simulink model "APP_MyApplication"  (R2018b)
settings: Solver=VariableStepDiscrete  StartTime=0.0  StopTime=10  RelTol=1e-3
PreLoadFcn:
  | if(exist('MBDS_ModelCallback', 'file')), MBDS_ModelCallback('PreLoad'); end;
PostLoadFcn:
  | if(exist('MBDS_ModelCallback', 'file')), MBDS_ModelCallback('PostLoad'); end;
InitFcn:
  | if(exist('MBDS_ModelCallback', 'file')), MBDS_ModelCallback('Init'); end;
StartFcn:
  | if(exist('MBDS_ModelCallback', 'file')), MBDS_ModelCallback('Start'); end;
StopFcn:
  | if(exist('MBDS_ModelCallback', 'file')), MBDS_ModelCallback('Stop'); end;
undefined symbols (not defined in the file): sigbuilder_block, Ts
libraries: KIBES_Signal x499, simulink x8
(part 6 of 10)

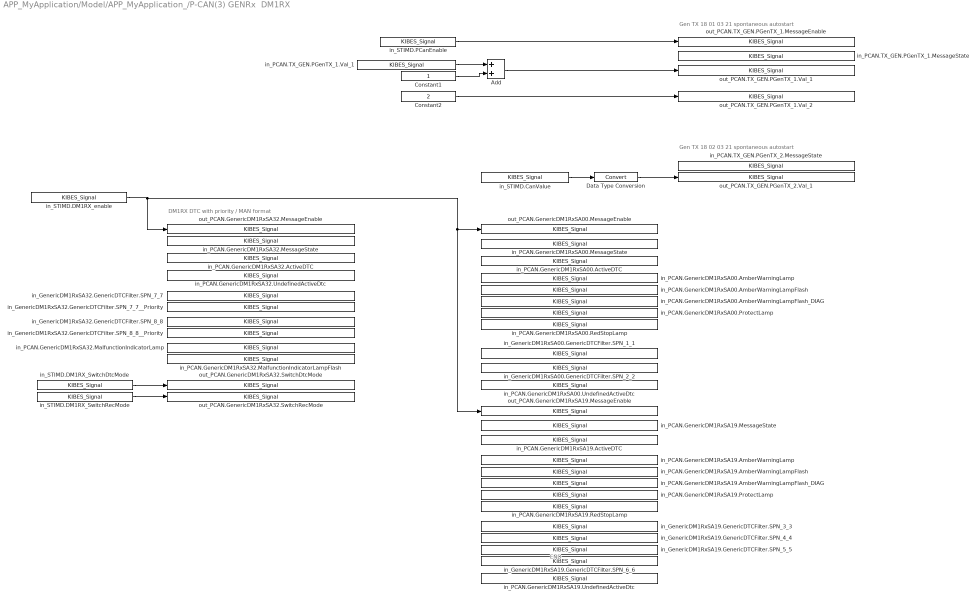
== system APP_MyApplication/Model/APP_MyApplication_/P-CAN(3) GENRx  DM1RX ==
  note: END
  note: Gen TX 18 01 03 21 spontaneous autostart
  note: Gen TX 18 02 03 21 spontaneous autostart
  note: DM1RX DTC with priority / MAN format
  Add : Sum  InitFcn=|  OutDataTypeStr=Inherit: Inherit via back propagation
      | if(exist('MBDS_BlockCallback', 'file'))
      |    MBDS_BlockCallback('Update', gcb);  
      | end
      settings: AttributesFormatString=Saturate: %<SaturateOnIntegerOverflow>
  Constant1 : Constant  InitFcn=|  OutDataTypeStr=uint8
      | if(exist('MBDS_BlockCallback', 'file'))
      |    MBDS_BlockCallback('Update', gcb);  
      | end
  Constant2 : Constant  InitFcn=|  Value=2  OutDataTypeStr=uint8
      | if(exist('MBDS_BlockCallback', 'file'))
      |    MBDS_BlockCallback('Update', gcb);  
      | end
  Data Type Conversion : DataTypeConversion  InitFcn=|  SaturateOnIntegerOverflow=on
      | try
      |    MBDS_BlockCallback('Update', gcb);
      | end
      settings: AttributesFormatString=Saturate: %<SaturateOnIntegerOverflow>
  in_GenericDM1RxSA00.GenericDTCFilter.SPN_1_1 : KIBES_Signal/KIBES_Signal  MBDS_LibraryBlock=on  DatabaseKey=293  SignalName=GenericDM1RxSA00.GenericDTCFilter.SPN_1_1  SymbolName=GenericDM1RxSA00_GenericDTCFilter_SPN_1_1_000293  DataType=boolean  Init=0  Slope=1  Bias=0  DataSize=1  fpDataType=boolean  BlockIOType=Inport  DeviceType=0
  in_GenericDM1RxSA00.GenericDTCFilter.SPN_2_2 : KIBES_Signal/KIBES_Signal  MBDS_LibraryBlock=on  DatabaseKey=294  SignalName=GenericDM1RxSA00.GenericDTCFilter.SPN_2_2  SymbolName=GenericDM1RxSA00_GenericDTCFilter_SPN_2_2_000294  DataType=boolean  Init=0  Slope=1  Bias=0  DataSize=1  fpDataType=boolean  BlockIOType=Inport  DeviceType=0
  in_GenericDM1RxSA19.GenericDTCFilter.SPN_3_3 : KIBES_Signal/KIBES_Signal  MBDS_LibraryBlock=on  DatabaseKey=290  SignalName=GenericDM1RxSA19.GenericDTCFilter.SPN_3_3  SymbolName=GenericDM1RxSA19_GenericDTCFilter_SPN_3_3_000290  DataType=boolean  Init=0  Slope=1  Bias=0  DataSize=1  fpDataType=boolean  BlockIOType=Inport  DeviceType=0
  in_GenericDM1RxSA19.GenericDTCFilter.SPN_4_4 : KIBES_Signal/KIBES_Signal  MBDS_LibraryBlock=on  DatabaseKey=291  SignalName=GenericDM1RxSA19.GenericDTCFilter.SPN_4_4  SymbolName=GenericDM1RxSA19_GenericDTCFilter_SPN_4_4_000291  DataType=boolean  Init=0  Slope=1  Bias=0  DataSize=1  fpDataType=boolean  BlockIOType=Inport  DeviceType=0
  in_GenericDM1RxSA19.GenericDTCFilter.SPN_5_5 : KIBES_Signal/KIBES_Signal  MBDS_LibraryBlock=on  DatabaseKey=296  SignalName=GenericDM1RxSA19.GenericDTCFilter.SPN_5_5  SymbolName=GenericDM1RxSA19_GenericDTCFilter_SPN_5_5_000296  DataType=boolean  Init=0  Slope=1  Bias=0  DataSize=1  fpDataType=boolean  BlockIOType=Inport  DeviceType=0
  in_GenericDM1RxSA19.GenericDTCFilter.SPN_6_6 : KIBES_Signal/KIBES_Signal  MBDS_LibraryBlock=on  DatabaseKey=303  SignalName=GenericDM1RxSA19.GenericDTCFilter.SPN_6_6  SymbolName=GenericDM1RxSA19_GenericDTCFilter_SPN_6_6_000303  DataType=boolean  Init=0  Slope=1  Bias=0  DataSize=1  fpDataType=boolean  BlockIOType=Inport  DeviceType=0
  in_GenericDM1RxSA32.GenericDTCFilter.SPN_7_7 : KIBES_Signal/KIBES_Signal  MBDS_LibraryBlock=on  DatabaseKey=592  SignalName=GenericDM1RxSA32.GenericDTCFilter.SPN_7_7  SymbolName=GenericDM1RxSA32_GenericDTCFilter_SPN_7_7_000592  DataType=boolean  Init=0  Slope=1  Bias=0  DataSize=1  fpDataType=boolean  BlockIOType=Inport  DeviceType=0
  in_GenericDM1RxSA32.GenericDTCFilter.SPN_7_7__Priority : KIBES_Signal/KIBES_Signal  MBDS_LibraryBlock=on  DatabaseKey=593  SignalName=GenericDM1RxSA32.GenericDTCFilter.SPN_7_7__Priority  SymbolName=GenericDM1RxSA32_GenericDTCFilter_SPN_7_7__Priority_000593  DataType=uint8  Init=0  Slope=1  Bias=0  DataSize=1  fpDataType=uint8  BlockIOType=Inport  DeviceType=0
  in_GenericDM1RxSA32.GenericDTCFilter.SPN_8_8 : KIBES_Signal/KIBES_Signal  MBDS_LibraryBlock=on  DatabaseKey=594  SignalName=GenericDM1RxSA32.GenericDTCFilter.SPN_8_8  SymbolName=GenericDM1RxSA32_GenericDTCFilter_SPN_8_8_000594  DataType=boolean  Init=0  Slope=1  Bias=0  DataSize=1  fpDataType=boolean  BlockIOType=Inport  DeviceType=0
  in_GenericDM1RxSA32.GenericDTCFilter.SPN_8_8__Priority : KIBES_Signal/KIBES_Signal  MBDS_LibraryBlock=on  DatabaseKey=595  SignalName=GenericDM1RxSA32.GenericDTCFilter.SPN_8_8__Priority  SymbolName=GenericDM1RxSA32_GenericDTCFilter_SPN_8_8__Priority_000595  DataType=uint8  Init=0  Slope=1  Bias=0  DataSize=1  fpDataType=uint8  BlockIOType=Inport  DeviceType=0
  in_PCAN.GenericDM1RxSA00.ActiveDTC : KIBES_Signal/KIBES_Signal  MBDS_LibraryBlock=on  DatabaseKey=274  SignalName=PCAN.GenericDM1RxSA00.ActiveDTC  SymbolName=PCAN_GenericDM1RxSA00_ActiveDTC_000274  DataType=boolean  Init=0  Slope=1  Bias=0  DataSize=1  fpDataType=boolean  BlockIOType=Inport  DeviceType=0
  in_PCAN.GenericDM1RxSA00.AmberWarningLamp : KIBES_Signal/KIBES_Signal  MBDS_LibraryBlock=on  DatabaseKey=275  SignalName=PCAN.GenericDM1RxSA00.AmberWarningLamp  SymbolName=PCAN_GenericDM1RxSA00_AmberWarningLamp_000275  DataType=boolean  Init=0  Slope=1  Bias=0  DataSize=1  fpDataType=boolean  BlockIOType=Inport  DeviceType=0
  in_PCAN.GenericDM1RxSA00.AmberWarningLampFlash : KIBES_Signal/KIBES_Signal  MBDS_LibraryBlock=on  DatabaseKey=276  SignalName=PCAN.GenericDM1RxSA00.AmberWarningLampFlash  SymbolName=PCAN_GenericDM1RxSA00_AmberWarningLampFlash_000276  DataType=uint8  Init=0  Slope=1  Bias=0  DataSize=1  fpDataType=uint8  BlockIOType=Inport  DeviceType=0
  in_PCAN.GenericDM1RxSA00.AmberWarningLampFlash_DIAG : KIBES_Signal/KIBES_Signal  MBDS_LibraryBlock=on  DatabaseKey=277  SignalName=PCAN.GenericDM1RxSA00.AmberWarningLampFlash_DIAG  SymbolName=PCAN_GenericDM1RxSA00_AmberWarningLampFlash_DIAG_000277  DataType=uint16  Init=1  Slope=1  Bias=0  DataSize=1  fpDataType=uint16  BlockIOType=Inport  DeviceType=0
  in_PCAN.GenericDM1RxSA00.MessageState : KIBES_Signal/KIBES_Signal  MBDS_LibraryBlock=on  DatabaseKey=279  SignalName=PCAN.GenericDM1RxSA00.MessageState  SymbolName=PCAN_GenericDM1RxSA00_MessageState_000279  DataType=uint16  Init=0  Slope=1  Bias=0  DataSize=1  fpDataType=uint16  BlockIOType=Inport  DeviceType=0
  in_PCAN.GenericDM1RxSA00.ProtectLamp : KIBES_Signal/KIBES_Signal  MBDS_LibraryBlock=on  DatabaseKey=280  SignalName=PCAN.GenericDM1RxSA00.ProtectLamp  SymbolName=PCAN_GenericDM1RxSA00_ProtectLamp_000280  DataType=boolean  Init=0  Slope=1  Bias=0  DataSize=1  fpDataType=boolean  BlockIOType=Inport  DeviceType=0
  in_PCAN.GenericDM1RxSA00.RedStopLamp : KIBES_Signal/KIBES_Signal  MBDS_LibraryBlock=on  DatabaseKey=281  SignalName=PCAN.GenericDM1RxSA00.RedStopLamp  SymbolName=PCAN_GenericDM1RxSA00_RedStopLamp_000281  DataType=boolean  Init=0  Slope=1  Bias=0  DataSize=1  fpDataType=boolean  BlockIOType=Inport  DeviceType=0
  in_PCAN.GenericDM1RxSA00.UndefinedActiveDtc : KIBES_Signal/KIBES_Signal  MBDS_LibraryBlock=on  DatabaseKey=403  SignalName=PCAN.GenericDM1RxSA00.UndefinedActiveDtc  SymbolName=PCAN_GenericDM1RxSA00_UndefinedActiveDtc_000403  DataType=boolean  Init=0  Slope=1  Bias=0  DataSize=1  fpDataType=boolean  BlockIOType=Inport  DeviceType=0
  in_PCAN.GenericDM1RxSA19.ActiveDTC : KIBES_Signal/KIBES_Signal  MBDS_LibraryBlock=on  DatabaseKey=282  SignalName=PCAN.GenericDM1RxSA19.ActiveDTC  SymbolName=PCAN_GenericDM1RxSA19_ActiveDTC_000282  DataType=boolean  Init=0  Slope=1  Bias=0  DataSize=1  fpDataType=boolean  BlockIOType=Inport  DeviceType=0
  in_PCAN.GenericDM1RxSA19.AmberWarningLamp : KIBES_Signal/KIBES_Signal  MBDS_LibraryBlock=on  DatabaseKey=283  SignalName=PCAN.GenericDM1RxSA19.AmberWarningLamp  SymbolName=PCAN_GenericDM1RxSA19_AmberWarningLamp_000283  DataType=boolean  Init=0  Slope=1  Bias=0  DataSize=1  fpDataType=boolean  BlockIOType=Inport  DeviceType=0
  in_PCAN.GenericDM1RxSA19.AmberWarningLampFlash : KIBES_Signal/KIBES_Signal  MBDS_LibraryBlock=on  DatabaseKey=284  SignalName=PCAN.GenericDM1RxSA19.AmberWarningLampFlash  SymbolName=PCAN_GenericDM1RxSA19_AmberWarningLampFlash_000284  DataType=uint8  Init=0  Slope=1  Bias=0  DataSize=1  fpDataType=uint8  BlockIOType=Inport  DeviceType=0
  in_PCAN.GenericDM1RxSA19.AmberWarningLampFlash_DIAG : KIBES_Signal/KIBES_Signal  MBDS_LibraryBlock=on  DatabaseKey=285  SignalName=PCAN.GenericDM1RxSA19.AmberWarningLampFlash_DIAG  SymbolName=PCAN_GenericDM1RxSA19_AmberWarningLampFlash_DIAG_000285  DataType=uint16  Init=1  Slope=1  Bias=0  DataSize=1  fpDataType=uint16  BlockIOType=Inport  DeviceType=0
  in_PCAN.GenericDM1RxSA19.MessageState : KIBES_Signal/KIBES_Signal  MBDS_LibraryBlock=on  DatabaseKey=287  SignalName=PCAN.GenericDM1RxSA19.MessageState  SymbolName=PCAN_GenericDM1RxSA19_MessageState_000287  DataType=uint16  Init=0  Slope=1  Bias=0  DataSize=1  fpDataType=uint16  BlockIOType=Inport  DeviceType=0
  in_PCAN.GenericDM1RxSA19.ProtectLamp : KIBES_Signal/KIBES_Signal  MBDS_LibraryBlock=on  DatabaseKey=288  SignalName=PCAN.GenericDM1RxSA19.ProtectLamp  SymbolName=PCAN_GenericDM1RxSA19_ProtectLamp_000288  DataType=boolean  Init=0  Slope=1  Bias=0  DataSize=1  fpDataType=boolean  BlockIOType=Inport  DeviceType=0
  in_PCAN.GenericDM1RxSA19.RedStopLamp : KIBES_Signal/KIBES_Signal  MBDS_LibraryBlock=on  DatabaseKey=289  SignalName=PCAN.GenericDM1RxSA19.RedStopLamp  SymbolName=PCAN_GenericDM1RxSA19_RedStopLamp_000289  DataType=boolean  Init=0  Slope=1  Bias=0  DataSize=1  fpDataType=boolean  BlockIOType=Inport  DeviceType=0
  in_PCAN.GenericDM1RxSA19.UndefinedActiveDtc : KIBES_Signal/KIBES_Signal  MBDS_LibraryBlock=on  DatabaseKey=404  SignalName=PCAN.GenericDM1RxSA19.UndefinedActiveDtc  SymbolName=PCAN_GenericDM1RxSA19_UndefinedActiveDtc_000404  DataType=boolean  Init=0  Slope=1  Bias=0  DataSize=1  fpDataType=boolean  BlockIOType=Inport  DeviceType=0
  in_PCAN.GenericDM1RxSA32.ActiveDTC : KIBES_Signal/KIBES_Signal  MBDS_LibraryBlock=on  DatabaseKey=588  SignalName=PCAN.GenericDM1RxSA32.ActiveDTC  SymbolName=PCAN_GenericDM1RxSA32_ActiveDTC_000588  DataType=boolean  Init=0  Slope=1  Bias=0  DataSize=1  fpDataType=boolean  BlockIOType=Inport  DeviceType=0
  in_PCAN.GenericDM1RxSA32.MalfunctionIndicatorLamp : KIBES_Signal/KIBES_Signal  MBDS_LibraryBlock=on  DatabaseKey=601  SignalName=PCAN.GenericDM1RxSA32.MalfunctionIndicatorLamp  SymbolName=PCAN_GenericDM1RxSA32_MalfunctionIndicatorLamp_000601  DataType=boolean  Init=0  Slope=1  Bias=0  DataSize=1  fpDataType=boolean  BlockIOType=Inport  DeviceType=0
  in_PCAN.GenericDM1RxSA32.MalfunctionIndicatorLampFlash : KIBES_Signal/KIBES_Signal  MBDS_LibraryBlock=on  DatabaseKey=602  SignalName=PCAN.GenericDM1RxSA32.MalfunctionIndicatorLampFlash  SymbolName=PCAN_GenericDM1RxSA32_MalfunctionIndicatorLampFlash_000602  DataType=uint8  Init=0  Slope=1  Bias=0  DataSize=1  fpDataType=uint8  BlockIOType=Inport  DeviceType=0
  in_PCAN.GenericDM1RxSA32.MessageState : KIBES_Signal/KIBES_Signal  MBDS_LibraryBlock=on  DatabaseKey=590  SignalName=PCAN.GenericDM1RxSA32.MessageState  SymbolName=PCAN_GenericDM1RxSA32_MessageState_000590  DataType=uint16  Init=0  Slope=1  Bias=0  DataSize=1  fpDataType=uint16  BlockIOType=Inport  DeviceType=0
  in_PCAN.GenericDM1RxSA32.UndefinedActiveDtc : KIBES_Signal/KIBES_Signal  MBDS_LibraryBlock=on  DatabaseKey=591  SignalName=PCAN.GenericDM1RxSA32.UndefinedActiveDtc  SymbolName=PCAN_GenericDM1RxSA32_UndefinedActiveDtc_000591  DataType=boolean  Init=0  Slope=1  Bias=0  DataSize=1  fpDataType=boolean  BlockIOType=Inport  DeviceType=0
  in_PCAN.TX_GEN.PGenTX_1.MessageState : KIBES_Signal/KIBES_Signal  MBDS_LibraryBlock=on  DatabaseKey=260  SignalName=PCAN.TX_GEN.PGenTX_1.MessageState  SymbolName=PCAN_TX_GEN_PGenTX_1_MessageState_000260  DataType=uint16  Init=0  Slope=1  Bias=0  DataSize=1  fpDataType=uint16  BlockIOType=Inport  DeviceType=0
  in_PCAN.TX_GEN.PGenTX_1.Val_1 : KIBES_Signal/KIBES_Signal  MBDS_LibraryBlock=on  DatabaseKey=261  SignalName=PCAN.TX_GEN.PGenTX_1.Val_1  SymbolName=PCAN_TX_GEN_PGenTX_1_Val_1_000261  DataType=uint8  Init=0  Slope=1  Bias=0  DataSize=1  fpDataType=uint8  BlockIOType=Inport  DeviceType=0
  in_PCAN.TX_GEN.PGenTX_2.MessageState : KIBES_Signal/KIBES_Signal  MBDS_LibraryBlock=on  DatabaseKey=577  SignalName=PCAN.TX_GEN.PGenTX_2.MessageState  SymbolName=PCAN_TX_GEN_PGenTX_2_MessageState_000577  DataType=uint16  Init=0  Slope=1  Bias=0  DataSize=1  fpDataType=uint16  BlockIOType=Inport  DeviceType=0
  in_STIMD.CanValue : KIBES_Signal/KIBES_Signal  MBDS_LibraryBlock=on  DatabaseKey=585  SignalName=STIMD.CanValue  SymbolName=STIMD_CanValue_000585  DataType=int32  Init=1  Slope=1  Bias=0  DataSize=1  fpDataType=int32  BlockIOType=Inport  DeviceType=2
  in_STIMD.DM1RX_SwitchDtcMode : KIBES_Signal/KIBES_Signal  MBDS_LibraryBlock=on  DatabaseKey=599  SignalName=STIMD.DM1RX_SwitchDtcMode  SymbolName=STIMD_DM1RX_SwitchDtcMode_000599  DataType=uint8  Init=0  Slope=1  Bias=0  DataSize=1  fpDataType=uint8  BlockIOType=Inport  DeviceType=2
  in_STIMD.DM1RX_SwitchRecMode : KIBES_Signal/KIBES_Signal  MBDS_LibraryBlock=on  DatabaseKey=600  SignalName=STIMD.DM1RX_SwitchRecMode  SymbolName=STIMD_DM1RX_SwitchRecMode_000600  DataType=uint8  Init=1  Slope=1  Bias=0  DataSize=1  fpDataType=uint8  BlockIOType=Inport  DeviceType=2
  in_STIMD.DM1RX_enable : KIBES_Signal/KIBES_Signal  MBDS_LibraryBlock=on  DatabaseKey=598  SignalName=STIMD.DM1RX_enable  SymbolName=STIMD_DM1RX_enable_000598  DataType=boolean  Init=1  Slope=1  Bias=0  DataSize=1  fpDataType=boolean  BlockIOType=Inport  DeviceType=2
  in_STIMD.PCanEnable : KIBES_Signal/KIBES_Signal  MBDS_LibraryBlock=on  DatabaseKey=497  SignalName=STIMD.PCanEnable  SymbolName=STIMD_PCanEnable_000497  DataType=boolean  Init=0  Slope=1  Bias=0  DataSize=1  fpDataType=boolean  BlockIOType=Inport  DeviceType=2
  out_PCAN.GenericDM1RxSA00.MessageEnable : KIBES_Signal/KIBES_Signal  MBDS_LibraryBlock=on  DatabaseKey=278  SignalName=PCAN.GenericDM1RxSA00.MessageEnable  SymbolName=PCAN_GenericDM1RxSA00_MessageEnable_000278  DataType=boolean  Init=0  Slope=1  Bias=0  DataSize=1  fpDataType=boolean  BlockIOType=Outport  DeviceType=0
  out_PCAN.GenericDM1RxSA19.MessageEnable : KIBES_Signal/KIBES_Signal  MBDS_LibraryBlock=on  DatabaseKey=286  SignalName=PCAN.GenericDM1RxSA19.MessageEnable  SymbolName=PCAN_GenericDM1RxSA19_MessageEnable_000286  DataType=boolean  Init=0  Slope=1  Bias=0  DataSize=1  fpDataType=boolean  BlockIOType=Outport  DeviceType=0
  out_PCAN.GenericDM1RxSA32.MessageEnable : KIBES_Signal/KIBES_Signal  MBDS_LibraryBlock=on  DatabaseKey=589  SignalName=PCAN.GenericDM1RxSA32.MessageEnable  SymbolName=PCAN_GenericDM1RxSA32_MessageEnable_000589  DataType=boolean  Init=0  Slope=1  Bias=0  DataSize=1  fpDataType=boolean  BlockIOType=Outport  DeviceType=0
  out_PCAN.GenericDM1RxSA32.SwitchDtcMode : KIBES_Signal/KIBES_Signal  MBDS_LibraryBlock=on  DatabaseKey=596  SignalName=PCAN.GenericDM1RxSA32.SwitchDtcMode  SymbolName=PCAN_GenericDM1RxSA32_SwitchDtcMode_000596  DataType=uint8  Init=0  Slope=1  Bias=0  DataSize=1  fpDataType=uint8  BlockIOType=Outport  DeviceType=0
  out_PCAN.GenericDM1RxSA32.SwitchRecMode : KIBES_Signal/KIBES_Signal  MBDS_LibraryBlock=on  DatabaseKey=597  SignalName=PCAN.GenericDM1RxSA32.SwitchRecMode  SymbolName=PCAN_GenericDM1RxSA32_SwitchRecMode_000597  DataType=uint8  Init=0  Slope=1  Bias=0  DataSize=1  fpDataType=uint8  BlockIOType=Outport  DeviceType=0
  out_PCAN.TX_GEN.PGenTX_1.MessageEnable : KIBES_Signal/KIBES_Signal  MBDS_LibraryBlock=on  DatabaseKey=259  SignalName=PCAN.TX_GEN.PGenTX_1.MessageEnable  SymbolName=PCAN_TX_GEN_PGenTX_1_MessageEnable_000259  DataType=boolean  Init=0  Slope=1  Bias=0  DataSize=1  fpDataType=boolean  BlockIOType=Outport  DeviceType=0
  out_PCAN.TX_GEN.PGenTX_1.Val_1 : KIBES_Signal/KIBES_Signal  MBDS_LibraryBlock=on  DatabaseKey=261  SignalName=PCAN.TX_GEN.PGenTX_1.Val_1  SymbolName=PCAN_TX_GEN_PGenTX_1_Val_1_000261  DataType=uint8  Init=0  Slope=1  Bias=0  DataSize=1  fpDataType=uint8  BlockIOType=Outport  DeviceType=0
  out_PCAN.TX_GEN.PGenTX_1.Val_2 : KIBES_Signal/KIBES_Signal  MBDS_LibraryBlock=on  DatabaseKey=262  SignalName=PCAN.TX_GEN.PGenTX_1.Val_2  SymbolName=PCAN_TX_GEN_PGenTX_1_Val_2_000262  DataType=uint8  Init=0  Slope=1  Bias=0  DataSize=1  fpDataType=uint8  BlockIOType=Outport  DeviceType=0
  out_PCAN.TX_GEN.PGenTX_2.Val_1 : KIBES_Signal/KIBES_Signal  MBDS_LibraryBlock=on  DatabaseKey=578  SignalName=PCAN.TX_GEN.PGenTX_2.Val_1  SymbolName=PCAN_TX_GEN_PGenTX_2_Val_1_000578  DataType=uint32  Init=0  Slope=1  Bias=0  DataSize=1  fpDataType=uint32  BlockIOType=Outport  DeviceType=0
  wires:
  in_STIMD.PCanEnable/1 -> out_PCAN.TX_GEN.PGenTX_1.MessageEnable/1
  Constant2/1 -> out_PCAN.TX_GEN.PGenTX_1.Val_2/1
  in_STIMD.DM1RX_enable/1 -> out_PCAN.GenericDM1RxSA19.MessageEnable/1, out_PCAN.GenericDM1RxSA00.MessageEnable/1, out_PCAN.GenericDM1RxSA32.MessageEnable/1
  Data Type Conversion/1 -> out_PCAN.TX_GEN.PGenTX_2.Val_1/1
  in_STIMD.CanValue/1 -> Data Type Conversion/1
  in_STIMD.DM1RX_SwitchDtcMode/1 -> out_PCAN.GenericDM1RxSA32.SwitchDtcMode/1
  in_STIMD.DM1RX_SwitchRecMode/1 -> out_PCAN.GenericDM1RxSA32.SwitchRecMode/1
  in_PCAN.TX_GEN.PGenTX_1.Val_1/1 -> Add/1
  Constant1/1 -> Add/2
  Add/1 -> out_PCAN.TX_GEN.PGenTX_1.Val_1/1

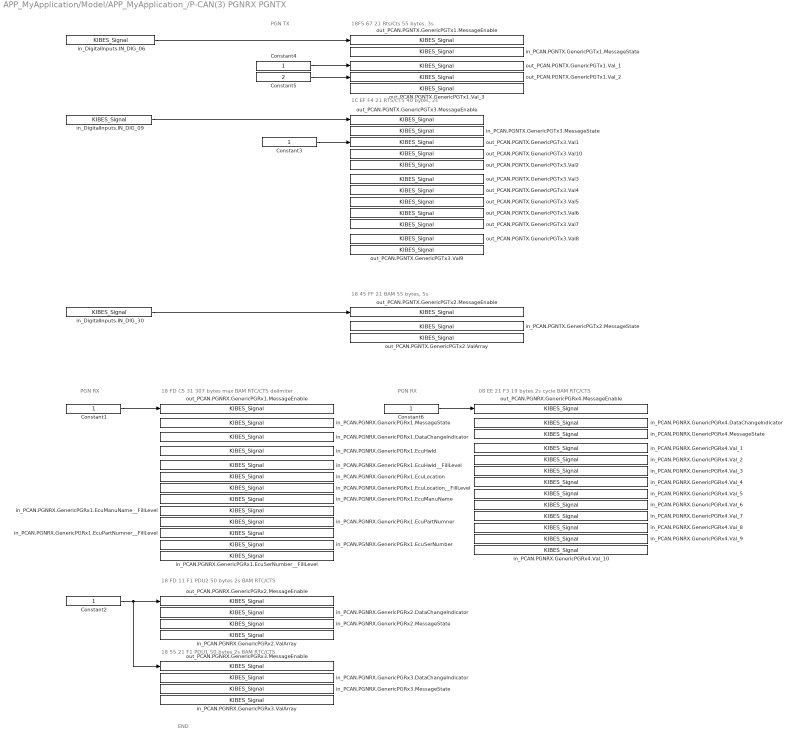
== system APP_MyApplication/Model/APP_MyApplication_/P-CAN(3) PGNRX PGNTX ==
  note: END
  note: 18 FD 11 F1 PDU2 50 bytes 2s BAM RTC/CTS
  note: 18 55 21 F1 PDU1 50 bytes 2s BAM RTC/CTS
  note: PGN TX
  note: PGN RX
  note: 18 45 FF 21 BAM 55 bytes, 5s
  note: 18F5 67 21 Rts/Cts 55 bytes, 3s
  note: 18 FD C5 31 307 bytes max BAM RTC/CTS delimiter
  note: 1C EF F4 21 RTS/CTS 40 bytes, 2s
  note: PGN RX
  note: 08 EE 21 F3 19 bytes 2s cycle BAM RTC/CTS
  Constant1 : Constant  InitFcn=|  OutDataTypeStr=boolean
      | if(exist('MBDS_BlockCallback', 'file'))
      |    MBDS_BlockCallback('Update', gcb);  
      | end
  Constant2 : Constant  InitFcn=|  OutDataTypeStr=boolean
      | if(exist('MBDS_BlockCallback', 'file'))
      |    MBDS_BlockCallback('Update', gcb);  
      | end
  Constant3 : Constant  InitFcn=|  OutDataTypeStr=uint32
      | if(exist('MBDS_BlockCallback', 'file'))
      |    MBDS_BlockCallback('Update', gcb);  
      | end
  Constant4 : Constant  InitFcn=|  OutDataTypeStr=uint8
      | if(exist('MBDS_BlockCallback', 'file'))
      |    MBDS_BlockCallback('Update', gcb);  
      | end
  Constant5 : Constant  InitFcn=|  Value=2  OutDataTypeStr=uint32
      | if(exist('MBDS_BlockCallback', 'file'))
      |    MBDS_BlockCallback('Update', gcb);  
      | end
  Constant6 : Constant  InitFcn=|  OutDataTypeStr=boolean
      | if(exist('MBDS_BlockCallback', 'file'))
      |    MBDS_BlockCallback('Update', gcb);  
      | end
  in_DigitalInputs.IN_DIG_06 : KIBES_Signal/KIBES_Signal  MBDS_LibraryBlock=on  DatabaseKey=463  SignalName=DigitalInputs.IN_DIG_06  SymbolName=DigitalInputs_IN_DIG_06_000463  DataType=boolean  Init=0  Slope=1  Bias=0  DataSize=1  fpDataType=boolean  BlockIOType=Inport  DeviceType=0
  in_DigitalInputs.IN_DIG_09 : KIBES_Signal/KIBES_Signal  MBDS_LibraryBlock=on  DatabaseKey=457  SignalName=DigitalInputs.IN_DIG_09  SymbolName=DigitalInputs_IN_DIG_09_000457  DataType=boolean  Init=0  Slope=1  Bias=0  DataSize=1  fpDataType=boolean  BlockIOType=Inport  DeviceType=0
  in_DigitalInputs.IN_DIG_30 : KIBES_Signal/KIBES_Signal  MBDS_LibraryBlock=on  DatabaseKey=480  SignalName=DigitalInputs.IN_DIG_30  SymbolName=DigitalInputs_IN_DIG_30_000480  DataType=boolean  Init=0  Slope=1  Bias=0  DataSize=1  fpDataType=boolean  BlockIOType=Inport  DeviceType=0
  in_PCAN.PGNRX.GenericPGRx1.DataChangeIndicator : KIBES_Signal/KIBES_Signal  MBDS_LibraryBlock=on  DatabaseKey=506  SignalName=PCAN.PGNRX.GenericPGRx1.DataChangeIndicator  SymbolName=PCAN_PGNRX_GenericPGRx1_DataChangeIndicator_000506  DataType=boolean  Init=0  Slope=1  Bias=0  DataSize=1  fpDataType=boolean  BlockIOType=Inport  DeviceType=0
  in_PCAN.PGNRX.GenericPGRx1.EcuHwId : KIBES_Signal/KIBES_Signal  MBDS_LibraryBlock=on  DatabaseKey=507  SignalName=PCAN.PGNRX.GenericPGRx1.EcuHwId  SymbolName=PCAN_PGNRX_GenericPGRx1_EcuHwId_000507  DataType=uint8  Init=[0 0 0 0 0 0 0 0 0 0 0 0 0 0 0 0 0 0 0 0 0 0 0 0 0 0 0 0 0 0 0 0 0 0 0 0 0 0 0 0 0 0 0 0 0 0 0 0 0 0 0 0 0 0 0 0 0 0 0 0 0]  Slope=1  Bias=0  DataSize=61  fpDataType=uint8  BlockIOType=Inport  DeviceType=0
  in_PCAN.PGNRX.GenericPGRx1.EcuHwId__FillLevel : KIBES_Signal/KIBES_Signal  MBDS_LibraryBlock=on  DatabaseKey=508  SignalName=PCAN.PGNRX.GenericPGRx1.EcuHwId__FillLevel  SymbolName=PCAN_PGNRX_GenericPGRx1_EcuHwId__FillLevel_000508  DataType=uint16  Init=0  Slope=1  Bias=0  DataSize=1  fpDataType=uint16  BlockIOType=Inport  DeviceType=0
  in_PCAN.PGNRX.GenericPGRx1.EcuLocation : KIBES_Signal/KIBES_Signal  MBDS_LibraryBlock=on  DatabaseKey=509  SignalName=PCAN.PGNRX.GenericPGRx1.EcuLocation  SymbolName=PCAN_PGNRX_GenericPGRx1_EcuLocation_000509  DataType=uint8  Init=[0,0,0,0,0,0,0,0,0,0,0,0,0,0,0,0,0,0,0,0,0,0,0,0,0,0,0,0,0,0,0,0,0,0,0,0,0,0,0,0,0,0,0,0,0,0,0,0,0,0,0,0,0,0,0,0,0,0,0,0,0]  Slope=1  Bias=0  DataSize=61  fpDataType=uint8  BlockIOType=Inport  DeviceType=0
  in_PCAN.PGNRX.GenericPGRx1.EcuLocation__FillLevel : KIBES_Signal/KIBES_Signal  MBDS_LibraryBlock=on  DatabaseKey=510  SignalName=PCAN.PGNRX.GenericPGRx1.EcuLocation__FillLevel  SymbolName=PCAN_PGNRX_GenericPGRx1_EcuLocation__FillLevel_000510  DataType=uint16  Init=0  Slope=1  Bias=0  DataSize=1  fpDataType=uint16  BlockIOType=Inport  DeviceType=0
  in_PCAN.PGNRX.GenericPGRx1.EcuManuName : KIBES_Signal/KIBES_Signal  MBDS_LibraryBlock=on  DatabaseKey=511  SignalName=PCAN.PGNRX.GenericPGRx1.EcuManuName  SymbolName=PCAN_PGNRX_GenericPGRx1_EcuManuName_000511  DataType=uint8  Init=[0 0 0 0 0 0 0 0 0 0 0 0 0 0 0 0 0 0 0 0 0 0 0 0 0 0 0 0 0 0 0 0 0 0 0 0 0 0 0 0 0 0 0 0 0 0 0 0 0 0 0 0 0 0 0 0 0 0 0 0 0]  Slope=1  Bias=0  DataSize=61  fpDataType=uint8  BlockIOType=Inport  DeviceType=0
  in_PCAN.PGNRX.GenericPGRx1.EcuManuName__FillLevel : KIBES_Signal/KIBES_Signal  MBDS_LibraryBlock=on  DatabaseKey=512  SignalName=PCAN.PGNRX.GenericPGRx1.EcuManuName__FillLevel  SymbolName=PCAN_PGNRX_GenericPGRx1_EcuManuName__FillLevel_000512  DataType=uint16  Init=0  Slope=1  Bias=0  DataSize=1  fpDataType=uint16  BlockIOType=Inport  DeviceType=0
  in_PCAN.PGNRX.GenericPGRx1.EcuPartNumner : KIBES_Signal/KIBES_Signal  MBDS_LibraryBlock=on  DatabaseKey=513  SignalName=PCAN.PGNRX.GenericPGRx1.EcuPartNumner  SymbolName=PCAN_PGNRX_GenericPGRx1_EcuPartNumner_000513  DataType=uint8  Init=[0 0 0 0 0 0 0 0 0 0 0 0 0 0 0 0 0 0 0 0 0 0 0 0 0 0 0 0 0 0 0 0 0 0 0 0 0 0 0 0 0 0 0 0 0 0 0 0 0 0 0 0 0 0 0 0 0 0 0 0 0]  Slope=1  Bias=0  DataSize=61  fpDataType=uint8  BlockIOType=Inport  DeviceType=0
  in_PCAN.PGNRX.GenericPGRx1.EcuPartNumner__FillLevel : KIBES_Signal/KIBES_Signal  MBDS_LibraryBlock=on  DatabaseKey=514  SignalName=PCAN.PGNRX.GenericPGRx1.EcuPartNumner__FillLevel  SymbolName=PCAN_PGNRX_GenericPGRx1_EcuPartNumner__FillLevel_000514  DataType=uint16  Init=0  Slope=1  Bias=0  DataSize=1  fpDataType=uint16  BlockIOType=Inport  DeviceType=0
  in_PCAN.PGNRX.GenericPGRx1.EcuSerNumber : KIBES_Signal/KIBES_Signal  MBDS_LibraryBlock=on  DatabaseKey=515  SignalName=PCAN.PGNRX.GenericPGRx1.EcuSerNumber  SymbolName=PCAN_PGNRX_GenericPGRx1_EcuSerNumber_000515  DataType=uint8  Init=[0 0 0 0 0 0 0 0 0 0 0 0 0 0 0 0 0 0 0 0 0 0 0 0 0 0 0 0 0 0 0 0 0 0 0 0 0 0 0 0 0 0 0 0 0 0 0 0 0 0 0 0 0 0 0 0 0 0 0 0 0]  Slope=1  Bias=0  DataSize=61  fpDataType=uint8  BlockIOType=Inport  DeviceType=0
  in_PCAN.PGNRX.GenericPGRx1.EcuSerNumber__FillLevel : KIBES_Signal/KIBES_Signal  MBDS_LibraryBlock=on  DatabaseKey=516  SignalName=PCAN.PGNRX.GenericPGRx1.EcuSerNumber__FillLevel  SymbolName=PCAN_PGNRX_GenericPGRx1_EcuSerNumber__FillLevel_000516  DataType=uint16  Init=0  Slope=1  Bias=0  DataSize=1  fpDataType=uint16  BlockIOType=Inport  DeviceType=0
  in_PCAN.PGNRX.GenericPGRx1.MessageState : KIBES_Signal/KIBES_Signal  MBDS_LibraryBlock=on  DatabaseKey=520  SignalName=PCAN.PGNRX.GenericPGRx1.MessageState  SymbolName=PCAN_PGNRX_GenericPGRx1_MessageState_000520  DataType=uint16  Init=0  Slope=1  Bias=0  DataSize=1  fpDataType=uint16  BlockIOType=Inport  DeviceType=0
  in_PCAN.PGNRX.GenericPGRx2.DataChangeIndicator : KIBES_Signal/KIBES_Signal  MBDS_LibraryBlock=on  DatabaseKey=521  SignalName=PCAN.PGNRX.GenericPGRx2.DataChangeIndicator  SymbolName=PCAN_PGNRX_GenericPGRx2_DataChangeIndicator_000521  DataType=boolean  Init=0  Slope=1  Bias=0  DataSize=1  fpDataType=boolean  BlockIOType=Inport  DeviceType=0
  in_PCAN.PGNRX.GenericPGRx2.MessageState : KIBES_Signal/KIBES_Signal  MBDS_LibraryBlock=on  DatabaseKey=523  SignalName=PCAN.PGNRX.GenericPGRx2.MessageState  SymbolName=PCAN_PGNRX_GenericPGRx2_MessageState_000523  DataType=uint16  Init=0  Slope=1  Bias=0  DataSize=1  fpDataType=uint16  BlockIOType=Inport  DeviceType=0
  in_PCAN.PGNRX.GenericPGRx2.ValArray : KIBES_Signal/KIBES_Signal  MBDS_LibraryBlock=on  DatabaseKey=524  SignalName=PCAN.PGNRX.GenericPGRx2.ValArray  SymbolName=PCAN_PGNRX_GenericPGRx2_ValArray_000524  DataType=uint8  Init=[0,0,0,0,0,0,0,0,0,0,0,0,0,0,0,0,0,0,0,0,0,0,0,0,0,0,0,0,0,0,0,0,0,0,0,0,0,0,0,0,0,0,0,0,0,0,0,0,0,0]  Slope=1  Bias=0  DataSize=50  fpDataType=uint8  BlockIOType=Inport  DeviceType=0
  in_PCAN.PGNRX.GenericPGRx3.DataChangeIndicator : KIBES_Signal/KIBES_Signal  MBDS_LibraryBlock=on  DatabaseKey=525  SignalName=PCAN.PGNRX.GenericPGRx3.DataChangeIndicator  SymbolName=PCAN_PGNRX_GenericPGRx3_DataChangeIndicator_000525  DataType=boolean  Init=0  Slope=1  Bias=0  DataSize=1  fpDataType=boolean  BlockIOType=Inport  DeviceType=0
  in_PCAN.PGNRX.GenericPGRx3.MessageState : KIBES_Signal/KIBES_Signal  MBDS_LibraryBlock=on  DatabaseKey=527  SignalName=PCAN.PGNRX.GenericPGRx3.MessageState  SymbolName=PCAN_PGNRX_GenericPGRx3_MessageState_000527  DataType=uint16  Init=0  Slope=1  Bias=0  DataSize=1  fpDataType=uint16  BlockIOType=Inport  DeviceType=0
  in_PCAN.PGNRX.GenericPGRx3.ValArray : KIBES_Signal/KIBES_Signal  MBDS_LibraryBlock=on  DatabaseKey=528  SignalName=PCAN.PGNRX.GenericPGRx3.ValArray  SymbolName=PCAN_PGNRX_GenericPGRx3_ValArray_000528  DataType=uint8  Init=[0,0,0,0,0,0,0,0,0,0,0,0,0,0,0,0,0,0,0,0,0,0,0,0,0,0,0,0,0,0,0,0,0,0,0,0,0,0,0,0,0,0,0,0,0,0,0,0,0,0]  Slope=1  Bias=0  DataSize=50  fpDataType=uint8  BlockIOType=Inport  DeviceType=0
  in_PCAN.PGNRX.GenericPGRx4.DataChangeIndicator : KIBES_Signal/KIBES_Signal  MBDS_LibraryBlock=on  DatabaseKey=562  SignalName=PCAN.PGNRX.GenericPGRx4.DataChangeIndicator  SymbolName=PCAN_PGNRX_GenericPGRx4_DataChangeIndicator_000562  DataType=boolean  Init=0  Slope=1  Bias=0  DataSize=1  fpDataType=boolean  BlockIOType=Inport  DeviceType=0
  in_PCAN.PGNRX.GenericPGRx4.MessageState : KIBES_Signal/KIBES_Signal  MBDS_LibraryBlock=on  DatabaseKey=564  SignalName=PCAN.PGNRX.GenericPGRx4.MessageState  SymbolName=PCAN_PGNRX_GenericPGRx4_MessageState_000564  DataType=uint16  Init=0  Slope=1  Bias=0  DataSize=1  fpDataType=uint16  BlockIOType=Inport  DeviceType=0
  in_PCAN.PGNRX.GenericPGRx4.Val_1 : KIBES_Signal/KIBES_Signal  MBDS_LibraryBlock=on  DatabaseKey=565  SignalName=PCAN.PGNRX.GenericPGRx4.Val_1  SymbolName=PCAN_PGNRX_GenericPGRx4_Val_1_000565  DataType=uint8  Init=0  Slope=1  Bias=0  DataSize=1  fpDataType=uint8  BlockIOType=Inport  DeviceType=0
  in_PCAN.PGNRX.GenericPGRx4.Val_10 : KIBES_Signal/KIBES_Signal  MBDS_LibraryBlock=on  DatabaseKey=566  SignalName=PCAN.PGNRX.GenericPGRx4.Val_10  SymbolName=PCAN_PGNRX_GenericPGRx4_Val_10_000566  DataType=uint32  Init=0  Slope=1  Bias=0  DataSize=1  fpDataType=uint32  BlockIOType=Inport  DeviceType=0
  in_PCAN.PGNRX.GenericPGRx4.Val_2 : KIBES_Signal/KIBES_Signal  MBDS_LibraryBlock=on  DatabaseKey=567  SignalName=PCAN.PGNRX.GenericPGRx4.Val_2  SymbolName=PCAN_PGNRX_GenericPGRx4_Val_2_000567  DataType=uint8  Init=0  Slope=1  Bias=0  DataSize=1  fpDataType=uint8  BlockIOType=Inport  DeviceType=0
  in_PCAN.PGNRX.GenericPGRx4.Val_3 : KIBES_Signal/KIBES_Signal  MBDS_LibraryBlock=on  DatabaseKey=568  SignalName=PCAN.PGNRX.GenericPGRx4.Val_3  SymbolName=PCAN_PGNRX_GenericPGRx4_Val_3_000568  DataType=boolean  Init=0  Slope=1  Bias=0  DataSize=1  fpDataType=boolean  BlockIOType=Inport  DeviceType=0
  in_PCAN.PGNRX.GenericPGRx4.Val_4 : KIBES_Signal/KIBES_Signal  MBDS_LibraryBlock=on  DatabaseKey=569  SignalName=PCAN.PGNRX.GenericPGRx4.Val_4  SymbolName=PCAN_PGNRX_GenericPGRx4_Val_4_000569  DataType=uint8  Init=0  Slope=1  Bias=0  DataSize=1  fpDataType=uint8  BlockIOType=Inport  DeviceType=0
  in_PCAN.PGNRX.GenericPGRx4.Val_5 : KIBES_Signal/KIBES_Signal  MBDS_LibraryBlock=on  DatabaseKey=570  SignalName=PCAN.PGNRX.GenericPGRx4.Val_5  SymbolName=PCAN_PGNRX_GenericPGRx4_Val_5_000570  DataType=uint8  Init=0  Slope=1  Bias=0  DataSize=1  fpDataType=uint8  BlockIOType=Inport  DeviceType=0
  in_PCAN.PGNRX.GenericPGRx4.Val_6 : KIBES_Signal/KIBES_Signal  MBDS_LibraryBlock=on  DatabaseKey=571  SignalName=PCAN.PGNRX.GenericPGRx4.Val_6  SymbolName=PCAN_PGNRX_GenericPGRx4_Val_6_000571  DataType=uint16  Init=0  Slope=1  Bias=0  DataSize=1  fpDataType=uint16  BlockIOType=Inport  DeviceType=0
  in_PCAN.PGNRX.GenericPGRx4.Val_7 : KIBES_Signal/KIBES_Signal  MBDS_LibraryBlock=on  DatabaseKey=572  SignalName=PCAN.PGNRX.GenericPGRx4.Val_7  SymbolName=PCAN_PGNRX_GenericPGRx4_Val_7_000572  DataType=uint16  Init=0  Slope=1  Bias=0  DataSize=1  fpDataType=uint16  BlockIOType=Inport  DeviceType=0
  in_PCAN.PGNRX.GenericPGRx4.Val_8 : KIBES_Signal/KIBES_Signal  MBDS_LibraryBlock=on  DatabaseKey=573  SignalName=PCAN.PGNRX.GenericPGRx4.Val_8  SymbolName=PCAN_PGNRX_GenericPGRx4_Val_8_000573  DataType=uint32  Init=0  Slope=1  Bias=0  DataSize=1  fpDataType=uint32  BlockIOType=Inport  DeviceType=0
  in_PCAN.PGNRX.GenericPGRx4.Val_9 : KIBES_Signal/KIBES_Signal  MBDS_LibraryBlock=on  DatabaseKey=574  SignalName=PCAN.PGNRX.GenericPGRx4.Val_9  SymbolName=PCAN_PGNRX_GenericPGRx4_Val_9_000574  DataType=uint32  Init=0  Slope=1  Bias=0  DataSize=1  fpDataType=uint32  BlockIOType=Inport  DeviceType=0
  in_PCAN.PGNTX.GenericPGTx1.MessageState : KIBES_Signal/KIBES_Signal  MBDS_LibraryBlock=on  DatabaseKey=501  SignalName=PCAN.PGNTX.GenericPGTx1.MessageState  SymbolName=PCAN_PGNTX_GenericPGTx1_MessageState_000501  DataType=uint16  Init=0  Slope=1  Bias=0  DataSize=1  fpDataType=uint16  BlockIOType=Inport  DeviceType=0
  in_PCAN.PGNTX.GenericPGTx2.MessageState : KIBES_Signal/KIBES_Signal  MBDS_LibraryBlock=on  DatabaseKey=530  SignalName=PCAN.PGNTX.GenericPGTx2.MessageState  SymbolName=PCAN_PGNTX_GenericPGTx2_MessageState_000530  DataType=uint16  Init=0  Slope=1  Bias=0  DataSize=1  fpDataType=uint16  BlockIOType=Inport  DeviceType=0
  in_PCAN.PGNTX.GenericPGTx3.MessageState : KIBES_Signal/KIBES_Signal  MBDS_LibraryBlock=on  DatabaseKey=551  SignalName=PCAN.PGNTX.GenericPGTx3.MessageState  SymbolName=PCAN_PGNTX_GenericPGTx3_MessageState_000551  DataType=uint16  Init=0  Slope=1  Bias=0  DataSize=1  fpDataType=uint16  BlockIOType=Inport  DeviceType=0
  out_PCAN.PGNRX.GenericPGRx1.MessageEnable : KIBES_Signal/KIBES_Signal  MBDS_LibraryBlock=on  DatabaseKey=519  SignalName=PCAN.PGNRX.GenericPGRx1.MessageEnable  SymbolName=PCAN_PGNRX_GenericPGRx1_MessageEnable_000519  DataType=boolean  Init=0  Slope=1  Bias=0  DataSize=1  fpDataType=boolean  BlockIOType=Outport  DeviceType=0
  out_PCAN.PGNRX.GenericPGRx2.MessageEnable : KIBES_Signal/KIBES_Signal  MBDS_LibraryBlock=on  DatabaseKey=522  SignalName=PCAN.PGNRX.GenericPGRx2.MessageEnable  SymbolName=PCAN_PGNRX_GenericPGRx2_MessageEnable_000522  DataType=boolean  Init=0  Slope=1  Bias=0  DataSize=1  fpDataType=boolean  BlockIOType=Outport  DeviceType=0
  out_PCAN.PGNRX.GenericPGRx3.MessageEnable : KIBES_Signal/KIBES_Signal  MBDS_LibraryBlock=on  DatabaseKey=526  SignalName=PCAN.PGNRX.GenericPGRx3.MessageEnable  SymbolName=PCAN_PGNRX_GenericPGRx3_MessageEnable_000526  DataType=boolean  Init=0  Slope=1  Bias=0  DataSize=1  fpDataType=boolean  BlockIOType=Outport  DeviceType=0
  out_PCAN.PGNRX.GenericPGRx4.MessageEnable : KIBES_Signal/KIBES_Signal  MBDS_LibraryBlock=on  DatabaseKey=563  SignalName=PCAN.PGNRX.GenericPGRx4.MessageEnable  SymbolName=PCAN_PGNRX_GenericPGRx4_MessageEnable_000563  DataType=boolean  Init=0  Slope=1  Bias=0  DataSize=1  fpDataType=boolean  BlockIOType=Outport  DeviceType=0
  out_PCAN.PGNTX.GenericPGTx1.MessageEnable : KIBES_Signal/KIBES_Signal  MBDS_LibraryBlock=on  DatabaseKey=500  SignalName=PCAN.PGNTX.GenericPGTx1.MessageEnable  SymbolName=PCAN_PGNTX_GenericPGTx1_MessageEnable_000500  DataType=boolean  Init=0  Slope=1  Bias=0  DataSize=1  fpDataType=boolean  BlockIOType=Outport  DeviceType=0
  out_PCAN.PGNTX.GenericPGTx1.Val_1 : KIBES_Signal/KIBES_Signal  MBDS_LibraryBlock=on  DatabaseKey=503  SignalName=PCAN.PGNTX.GenericPGTx1.Val_1  SymbolName=PCAN_PGNTX_GenericPGTx1_Val_1_000503  DataType=uint8  Init=0  Slope=1  Bias=0  DataSize=1  fpDataType=uint8  BlockIOType=Outport  DeviceType=0
  out_PCAN.PGNTX.GenericPGTx1.Val_2 : KIBES_Signal/KIBES_Signal  MBDS_LibraryBlock=on  DatabaseKey=504  SignalName=PCAN.PGNTX.GenericPGTx1.Val_2  SymbolName=PCAN_PGNTX_GenericPGTx1_Val_2_000504  DataType=uint32  Init=0  Slope=1  Bias=0  DataSize=1  fpDataType=uint32  BlockIOType=Outport  DeviceType=0
  out_PCAN.PGNTX.GenericPGTx1.Val_3 : KIBES_Signal/KIBES_Signal  MBDS_LibraryBlock=on  DatabaseKey=505  SignalName=PCAN.PGNTX.GenericPGTx1.Val_3  SymbolName=PCAN_PGNTX_GenericPGTx1_Val_3_000505  DataType=uint8  Init=[0,0,0,0,0,0,0,0,0,0,0,0,0,0,0,0,0,0,0,0,0,0,0,0,0,0,0,0,0,0,0,0,0,0,0,0,0,0,0,0,0,0,0,0,0,0,0,0,0,0]  Slope=1  Bias=0  DataSize=50  fpDataType=uint8  BlockIOType=Outport  DeviceType=0
  out_PCAN.PGNTX.GenericPGTx2.MessageEnable : KIBES_Signal/KIBES_Signal  MBDS_LibraryBlock=on  DatabaseKey=529  SignalName=PCAN.PGNTX.GenericPGTx2.MessageEnable  SymbolName=PCAN_PGNTX_GenericPGTx2_MessageEnable_000529  DataType=boolean  Init=0  Slope=1  Bias=0  DataSize=1  fpDataType=boolean  BlockIOType=Outport  DeviceType=0
  out_PCAN.PGNTX.GenericPGTx2.ValArray : KIBES_Signal/KIBES_Signal  MBDS_LibraryBlock=on  DatabaseKey=531  SignalName=PCAN.PGNTX.GenericPGTx2.ValArray  SymbolName=PCAN_PGNTX_GenericPGTx2_ValArray_000531  DataType=uint8  Init=[0,0,0,0,0,0,0,0,0,0,0,0,0,0,0,0,0,0,0,0]  Slope=1  Bias=0  DataSize=20  fpDataType=uint8  BlockIOType=Outport  DeviceType=0
  out_PCAN.PGNTX.GenericPGTx3.MessageEnable : KIBES_Signal/KIBES_Signal  MBDS_LibraryBlock=on  DatabaseKey=550  SignalName=PCAN.PGNTX.GenericPGTx3.MessageEnable  SymbolName=PCAN_PGNTX_GenericPGTx3_MessageEnable_000550  DataType=boolean  Init=0  Slope=1  Bias=0  DataSize=1  fpDataType=boolean  BlockIOType=Outport  DeviceType=0
  out_PCAN.PGNTX.GenericPGTx3.Val1 : KIBES_Signal/KIBES_Signal  MBDS_LibraryBlock=on  DatabaseKey=552  SignalName=PCAN.PGNTX.GenericPGTx3.Val1  SymbolName=PCAN_PGNTX_GenericPGTx3_Val1_000552  DataType=uint32  Init=0  Slope=1  Bias=0  DataSize=1  fpDataType=uint32  BlockIOType=Outport  DeviceType=0
  out_PCAN.PGNTX.GenericPGTx3.Val10 : KIBES_Signal/KIBES_Signal  MBDS_LibraryBlock=on  DatabaseKey=553  SignalName=PCAN.PGNTX.GenericPGTx3.Val10  SymbolName=PCAN_PGNTX_GenericPGTx3_Val10_000553  DataType=uint32  Init=0  Slope=1  Bias=0  DataSize=1  fpDataType=uint32  BlockIOType=Outport  DeviceType=0
  out_PCAN.PGNTX.GenericPGTx3.Val2 : KIBES_Signal/KIBES_Signal  MBDS_LibraryBlock=on  DatabaseKey=554  SignalName=PCAN.PGNTX.GenericPGTx3.Val2  SymbolName=PCAN_PGNTX_GenericPGTx3_Val2_000554  DataType=uint32  Init=0  Slope=1  Bias=0  DataSize=1  fpDataType=uint32  BlockIOType=Outport  DeviceType=0
  out_PCAN.PGNTX.GenericPGTx3.Val3 : KIBES_Signal/KIBES_Signal  MBDS_LibraryBlock=on  DatabaseKey=555  SignalName=PCAN.PGNTX.GenericPGTx3.Val3  SymbolName=PCAN_PGNTX_GenericPGTx3_Val3_000555  DataType=uint32  Init=0  Slope=1  Bias=0  DataSize=1  fpDataType=uint32  BlockIOType=Outport  DeviceType=0
  out_PCAN.PGNTX.GenericPGTx3.Val4 : KIBES_Signal/KIBES_Signal  MBDS_LibraryBlock=on  DatabaseKey=556  SignalName=PCAN.PGNTX.GenericPGTx3.Val4  SymbolName=PCAN_PGNTX_GenericPGTx3_Val4_000556  DataType=uint32  Init=0  Slope=1  Bias=0  DataSize=1  fpDataType=uint32  BlockIOType=Outport  DeviceType=0
  out_PCAN.PGNTX.GenericPGTx3.Val5 : KIBES_Signal/KIBES_Signal  MBDS_LibraryBlock=on  DatabaseKey=557  SignalName=PCAN.PGNTX.GenericPGTx3.Val5  SymbolName=PCAN_PGNTX_GenericPGTx3_Val5_000557  DataType=uint32  Init=0  Slope=1  Bias=0  DataSize=1  fpDataType=uint32  BlockIOType=Outport  DeviceType=0
  out_PCAN.PGNTX.GenericPGTx3.Val6 : KIBES_Signal/KIBES_Signal  MBDS_LibraryBlock=on  DatabaseKey=558  SignalName=PCAN.PGNTX.GenericPGTx3.Val6  SymbolName=PCAN_PGNTX_GenericPGTx3_Val6_000558  DataType=uint32  Init=0  Slope=1  Bias=0  DataSize=1  fpDataType=uint32  BlockIOType=Outport  DeviceType=0
  out_PCAN.PGNTX.GenericPGTx3.Val7 : KIBES_Signal/KIBES_Signal  MBDS_LibraryBlock=on  DatabaseKey=559  SignalName=PCAN.PGNTX.GenericPGTx3.Val7  SymbolName=PCAN_PGNTX_GenericPGTx3_Val7_000559  DataType=uint32  Init=0  Slope=1  Bias=0  DataSize=1  fpDataType=uint32  BlockIOType=Outport  DeviceType=0
  out_PCAN.PGNTX.GenericPGTx3.Val8 : KIBES_Signal/KIBES_Signal  MBDS_LibraryBlock=on  DatabaseKey=560  SignalName=PCAN.PGNTX.GenericPGTx3.Val8  SymbolName=PCAN_PGNTX_GenericPGTx3_Val8_000560  DataType=uint32  Init=0  Slope=1  Bias=0  DataSize=1  fpDataType=uint32  BlockIOType=Outport  DeviceType=0
  out_PCAN.PGNTX.GenericPGTx3.Val9 : KIBES_Signal/KIBES_Signal  MBDS_LibraryBlock=on  DatabaseKey=561  SignalName=PCAN.PGNTX.GenericPGTx3.Val9  SymbolName=PCAN_PGNTX_GenericPGTx3_Val9_000561  DataType=uint32  Init=0  Slope=1  Bias=0  DataSize=1  fpDataType=uint32  BlockIOType=Outport  DeviceType=0
  wires:
  in_DigitalInputs.IN_DIG_06/1 -> out_PCAN.PGNTX.GenericPGTx1.MessageEnable/1
  Constant4/1 -> out_PCAN.PGNTX.GenericPGTx1.Val_1/1
  Constant5/1 -> out_PCAN.PGNTX.GenericPGTx1.Val_2/1
  Constant1/1 -> out_PCAN.PGNRX.GenericPGRx1.MessageEnable/1
  Constant2/1 -> out_PCAN.PGNRX.GenericPGRx3.MessageEnable/1, out_PCAN.PGNRX.GenericPGRx2.MessageEnable/1
  in_DigitalInputs.IN_DIG_30/1 -> out_PCAN.PGNTX.GenericPGTx2.MessageEnable/1
  Constant3/1 -> out_PCAN.PGNTX.GenericPGTx3.Val1/1
  in_DigitalInputs.IN_DIG_09/1 -> out_PCAN.PGNTX.GenericPGTx3.MessageEnable/1
  Constant6/1 -> out_PCAN.PGNRX.GenericPGRx4.MessageEnable/1

== system APP_MyApplication/Model/APP_MyApplication_/RAM Device DataType ==
  Data Type Conversion : DataTypeConversion  InitFcn=|  SaturateOnIntegerOverflow=on
      | try
      |    MBDS_BlockCallback('Update', gcb);
      | end
      settings: AttributesFormatString=Saturate: %<SaturateOnIntegerOverflow>
  Data Type Conversion1 : DataTypeConversion  InitFcn=|  SaturateOnIntegerOverflow=on
      | try
      |    MBDS_BlockCallback('Update', gcb);
      | end
      settings: AttributesFormatString=Saturate: %<SaturateOnIntegerOverflow>
  in_STIMD.TypeReal : KIBES_Signal/KIBES_Signal  MBDS_LibraryBlock=on  DatabaseKey=587  SignalName=STIMD.TypeReal  SymbolName=STIMD_TypeReal_000587  DataType=single  Init=234.5678  Slope=1  Bias=0  DataSize=1  fpDataType=single  BlockIOType=Inport  DeviceType=2
  in_STIMD.TypeTest : KIBES_Signal/KIBES_Signal  MBDS_LibraryBlock=on  DatabaseKey=583  SignalName=STIMD.TypeTest  SymbolName=STIMD_TypeTest_000583  DataType=int32  Init=0  Slope=1  Bias=0  DataSize=1  fpDataType=int32  BlockIOType=Inport  DeviceType=2
  out_RAMDevice.TypeDINT : KIBES_Signal/KIBES_Signal  MBDS_LibraryBlock=on  DatabaseKey=580  SignalName=RAMDevice.TypeDINT  SymbolName=RAMDevice_TypeDINT_000580  DataType=int32  Init=0  Slope=1  Bias=0  DataSize=1  fpDataType=int32  BlockIOType=Outport  DeviceType=0
  out_RAMDevice.TypeINT : KIBES_Signal/KIBES_Signal  MBDS_LibraryBlock=on  DatabaseKey=581  SignalName=RAMDevice.TypeINT  SymbolName=RAMDevice_TypeINT_000581  DataType=int16  Init=0  Slope=1  Bias=0  DataSize=1  fpDataType=int16  BlockIOType=Outport  DeviceType=0
  out_RAMDevice.TypeREAL : KIBES_Signal/KIBES_Signal  MBDS_LibraryBlock=on  DatabaseKey=586  SignalName=RAMDevice.TypeREAL  SymbolName=RAMDevice_TypeREAL_000586  DataType=single  Init=0.0  Slope=1  Bias=0  DataSize=1  fpDataType=single  BlockIOType=Outport  DeviceType=0
  out_RAMDevice.TypeSINT : KIBES_Signal/KIBES_Signal  MBDS_LibraryBlock=on  DatabaseKey=582  SignalName=RAMDevice.TypeSINT  SymbolName=RAMDevice_TypeSINT_000582  DataType=int8  Init=0  Slope=1  Bias=0  DataSize=1  fpDataType=int8  BlockIOType=Outport  DeviceType=0
  wires:
  in_STIMD.TypeTest/1 -> Data Type Conversion1/1, Data Type Conversion/1, out_RAMDevice.TypeDINT/1
  Data Type Conversion/1 -> out_RAMDevice.TypeINT/1
  Data Type Conversion1/1 -> out_RAMDevice.TypeSINT/1
  in_STIMD.TypeReal/1 -> out_RAMDevice.TypeREAL/1
